simulink model "robot_rk"  (R2014b)
settings: Solver=ode45  StartTime=0.0  StopTime=10  FixedStep=1e-4  RelTol=1e-3
values from neighbouring files (symbols this model uses):
  robot_floor_friction_coeff = 0.6    [robot_init.m]
  robot_floor_position_gain = -1e5    (= -100000)    [robot_init.m]
  robot_floor_speed_gain = -1e3    (= -1000)    [robot_init.m]
  robot_gravity = [0 0 -9.80665]    [robot_init.m]
undefined symbols (not defined in the file or in its folder): CM730_acc_center, CM730_acc_gain, CM730_default, CM730_gyro_center, CM730_gyro_gain, CM730_sample_time, FSR_max, FSR_no_load, FSR_sample_time, FSR_scale, MX28_default, MX28_inertia, MX28_Te, X, Y, Z
libraries: sm_lib x158, fl_lib x128, nesl_utility x77
(part 4 of 6)

== system robot_rk/Right Leg/Right Ankle Pitch (15) ==
  Inertia : sm_lib/Body Elements/Inertia  InertiaType=Custom  Mass=1  MassUnits=g  CenterOfMass=[0 0 0]  CenterOfMassUnits=m  MomentsOfInertia=[0 0 MX28_inertia]  MomentsOfInertiaUnits=kg*m^2  ProductsOfInertia=[0 0 0]  ProductsOfInertiaUnits=kg*m^2  BlockFunction=simmechanics.library.body_elements.inertia
  MX28 Command : DataStoreRead  DataStoreName=MX28_ID15  SampleTime=MX28_Te  DataStoreElements=MX28_ID15.CW_angle_limit#MX28_ID15.CCW_angle_limit#MX28_ID15.torque_enable#MX28_ID15.D_gain#MX28_ID15.I_gain#MX28_ID15.P_gain#MX28_ID15.goal_position#MX28_ID15.moving_speed#MX28_ID15.torque_limit
  MX28 State : DataStoreWrite  DataStoreName=MX28_ID15  DataStoreElements=MX28_ID15.present_position#MX28_ID15.present_speed#MX28_ID15.present_load#MX28_ID15.moving#MX28_ID15.pwm
  Model : ModelReference  ModelNameDialog=MX28.slx  SimulationMode=Normal  ModelReferenceVersion=1.66  CopyOfModelName=MX28.slx  DefaultDataLogging=on
  Position converter : nesl_utility/PS-Simulink Converter  PhysicalDomain=network_engine_domain  SubClassName=ps_output  LeftPortType=input  RightPortType=output  PseudoPeriodic=off  Frequencies=[]  Unit=rad  AffineConversion=off
  Revolute Joint : sm_lib/Joints/Revolute Joint  SenseConstraintForce=off  SenseConstraintForceX=off  SenseConstraintForceY=off  SenseConstraintForceZ=off  SenseConstraintTorque=off  SenseConstraintTorqueX=off  SenseConstraintTorqueY=off  SenseConstraintTorqueZ=off  SenseTotalForce=off  SenseTotalForceX=off  SenseTotalForceY=off  SenseTotalForceZ=off  SenseTotalTorque=off  SenseTotalTorqueX=off  SenseTotalTorqueY=off  SenseTotalTorqueZ=off  CompositeWrenchDir=FollowerOnBase  CompositeWrenchFrame=BaseFrame  EquilibriumPosition=0  EquilibriumPositionUnits=deg  SpringStiffness=0  SpringStiffnessUnits=N*m/deg  DampingCoefficient=MX28_lub_friction  DampingCoefficientUnits=N*m/(rad/s)  TorqueActuationMode=InputTorque  MotionActuationMode=ComputedMotion  SensePosition=on  SenseVelocity=on  SenseAcceleration=off  SenseTorqueForce=off  PositionTargetValue=MX28_init_position  PositionTargetValueUnits=rad  PositionTargetSpecify=on  PositionTargetPriority=High  VelocityTargetValue=MX28_init_speed  VelocityTargetValueUnits=rad/s  VelocityTargetSpecify=on  VelocityTargetPriority=High  BlockFunction=simmechanics.library.joints.revolute_joint
  Speed converter : nesl_utility/PS-Simulink Converter  PhysicalDomain=network_engine_domain  SubClassName=ps_output  LeftPortType=input  RightPortType=output  PseudoPeriodic=off  Frequencies=[]  Unit=rad/s  AffineConversion=off
  Torque converter : nesl_utility/Simulink-PS Converter  PhysicalDomain=network_engine_domain  SubClassName=ps_input  LeftPortType=input  RightPortType=output  PseudoPeriodic=off  Frequencies=[]  NoiseDistribution=none  NoiseParameters=[]  Unit=N*m  AffineConversion=off  InputFiltering=off  SimscapeFilterOrder=1  InputFilterTimeConstant=0.001  UdotUserProvided=1
  Base : PMIOPort  Port=1  Side=Left
  Axis : PMIOPort  Port=2  Side=Right
  wires:
  Model/4 -> MX28 State/3
  Model/2 -> MX28 State/1
  Model/5 -> MX28 State/4
  Model/3 -> MX28 State/2
  MX28 Command/3 -> Model/5
  MX28 Command/6 -> Model/8
  MX28 Command/4 -> Model/6
  MX28 Command/5 -> Model/7
  MX28 Command/7 -> Model/9
  MX28 Command/2 -> Model/4
  MX28 Command/1 -> Model/3
  Position converter/1 -> Model/2
  Speed converter/1 -> Model/1
  Model/1 -> Torque converter/1
  Model/6 -> MX28 State/5
  MX28 Command/8 -> Model/10
  MX28 Command/9 -> Model/11
  connections:
  Axis/RConn1 -- Revolute Joint/RConn1 -- Inertia/RConn1
  Revolute Joint/LConn1 -- Base/RConn1
  Revolute Joint/RConn3 -- Speed converter/LConn1
  Revolute Joint/RConn2 -- Position converter/LConn1
  Revolute Joint/LConn2 -- Torque converter/RConn1

== system robot_rk/Right Leg/Right Ankle Roll (17) ==
  Inertia : sm_lib/Body Elements/Inertia  InertiaType=Custom  Mass=1  MassUnits=g  CenterOfMass=[0 0 0]  CenterOfMassUnits=m  MomentsOfInertia=[0 0 MX28_inertia]  MomentsOfInertiaUnits=kg*m^2  ProductsOfInertia=[0 0 0]  ProductsOfInertiaUnits=kg*m^2  BlockFunction=simmechanics.library.body_elements.inertia
  MX28 Command : DataStoreRead  DataStoreName=MX28_ID17  SampleTime=MX28_Te  DataStoreElements=MX28_ID17.CW_angle_limit#MX28_ID17.CCW_angle_limit#MX28_ID17.torque_enable#MX28_ID17.D_gain#MX28_ID17.I_gain#MX28_ID17.P_gain#MX28_ID17.goal_position#MX28_ID17.moving_speed#MX28_ID17.torque_limit
  MX28 State : DataStoreWrite  DataStoreName=MX28_ID17  DataStoreElements=MX28_ID17.present_position#MX28_ID17.present_speed#MX28_ID17.present_load#MX28_ID17.moving#MX28_ID17.pwm
  Model : ModelReference  ModelNameDialog=MX28.slx  SimulationMode=Normal  ModelReferenceVersion=1.66  CopyOfModelName=MX28.slx  DefaultDataLogging=on
  Position converter : nesl_utility/PS-Simulink Converter  PhysicalDomain=network_engine_domain  SubClassName=ps_output  LeftPortType=input  RightPortType=output  PseudoPeriodic=off  Frequencies=[]  Unit=rad  AffineConversion=off
  Revolute Joint : sm_lib/Joints/Revolute Joint  SenseConstraintForce=off  SenseConstraintForceX=off  SenseConstraintForceY=off  SenseConstraintForceZ=off  SenseConstraintTorque=off  SenseConstraintTorqueX=off  SenseConstraintTorqueY=off  SenseConstraintTorqueZ=off  SenseTotalForce=off  SenseTotalForceX=off  SenseTotalForceY=off  SenseTotalForceZ=off  SenseTotalTorque=off  SenseTotalTorqueX=off  SenseTotalTorqueY=off  SenseTotalTorqueZ=off  CompositeWrenchDir=FollowerOnBase  CompositeWrenchFrame=BaseFrame  EquilibriumPosition=0  EquilibriumPositionUnits=deg  SpringStiffness=0  SpringStiffnessUnits=N*m/deg  DampingCoefficient=MX28_lub_friction  DampingCoefficientUnits=N*m/(rad/s)  TorqueActuationMode=InputTorque  MotionActuationMode=ComputedMotion  SensePosition=on  SenseVelocity=on  SenseAcceleration=off  SenseTorqueForce=off  PositionTargetValue=MX28_init_position  PositionTargetValueUnits=rad  PositionTargetSpecify=on  PositionTargetPriority=High  VelocityTargetValue=MX28_init_speed  VelocityTargetValueUnits=rad/s  VelocityTargetSpecify=on  VelocityTargetPriority=High  BlockFunction=simmechanics.library.joints.revolute_joint
  Speed converter : nesl_utility/PS-Simulink Converter  PhysicalDomain=network_engine_domain  SubClassName=ps_output  LeftPortType=input  RightPortType=output  PseudoPeriodic=off  Frequencies=[]  Unit=rad/s  AffineConversion=off
  Torque converter : nesl_utility/Simulink-PS Converter  PhysicalDomain=network_engine_domain  SubClassName=ps_input  LeftPortType=input  RightPortType=output  PseudoPeriodic=off  Frequencies=[]  NoiseDistribution=none  NoiseParameters=[]  Unit=N*m  AffineConversion=off  InputFiltering=off  SimscapeFilterOrder=1  InputFilterTimeConstant=0.001  UdotUserProvided=1
  Base : PMIOPort  Port=1  Side=Left
  Axis : PMIOPort  Port=2  Side=Right
  wires:
  Model/4 -> MX28 State/3
  Model/2 -> MX28 State/1
  Model/5 -> MX28 State/4
  Model/3 -> MX28 State/2
  MX28 Command/3 -> Model/5
  MX28 Command/6 -> Model/8
  MX28 Command/4 -> Model/6
  MX28 Command/5 -> Model/7
  MX28 Command/7 -> Model/9
  MX28 Command/2 -> Model/4
  MX28 Command/1 -> Model/3
  Position converter/1 -> Model/2
  Speed converter/1 -> Model/1
  Model/1 -> Torque converter/1
  Model/6 -> MX28 State/5
  MX28 Command/8 -> Model/10
  MX28 Command/9 -> Model/11
  connections:
  Axis/RConn1 -- Revolute Joint/RConn1 -- Inertia/RConn1
  Revolute Joint/LConn1 -- Base/RConn1
  Revolute Joint/RConn3 -- Speed converter/LConn1
  Revolute Joint/RConn2 -- Position converter/LConn1
  Revolute Joint/LConn2 -- Torque converter/RConn1

== system robot_rk/Right Leg/Right Foot ==
  Right Foot Axis to Back Left : sm_lib/Frames and Transforms/Rigid Transform  TranslationMethod=Cartesian  TranslationLengthUnit=mm  TranslationStandardAxis=+Z  TranslationStandardOffset=0  TranslationCartesianOffset=[-14.5 33.5 -28.9]  TranslationROffset=0  TranslationROffsetUnits=m  TranslationZOffset=0  TranslationZOffsetUnits=m  TranslationThetaOffset=0  TranslationThetaOffsetUnits=deg  RotationMethod=AlignedAxes  RotationAngleUnits=deg  RotationStandardAxis=+Z  RotationAngle=0.0  RotationArbitraryAxis=[0 0 1]  FollAlignAxisA=+X  BaseAlignAxisA=-X  FollAlignAxisB=+Z  BaseAlignAxisB=-Y  RotationMatrix=[1 0 0; 0 1 0; 0 0 1]  BlockFunction=simmechanics.library.frames_transforms.rigid_transform
  Right Foot Axis to Back Right : sm_lib/Frames and Transforms/Rigid Transform  TranslationMethod=Cartesian  TranslationLengthUnit=mm  TranslationStandardAxis=+Z  TranslationStandardOffset=0  TranslationCartesianOffset=[35.5 33.5 -28.9]  TranslationROffset=0  TranslationROffsetUnits=m  TranslationZOffset=0  TranslationZOffsetUnits=m  TranslationThetaOffset=0  TranslationThetaOffsetUnits=deg  RotationMethod=AlignedAxes  RotationAngleUnits=deg  RotationStandardAxis=+Z  RotationAngle=0.0  RotationArbitraryAxis=[0 0 1]  FollAlignAxisA=+X  BaseAlignAxisA=-X  FollAlignAxisB=+Z  BaseAlignAxisB=-Y  RotationMatrix=[1 0 0; 0 1 0; 0 0 1]  BlockFunction=simmechanics.library.frames_transforms.rigid_transform
  Right Foot Axis to Front Left : sm_lib/Frames and Transforms/Rigid Transform  TranslationMethod=Cartesian  TranslationLengthUnit=mm  TranslationStandardAxis=+Z  TranslationStandardOffset=0  TranslationCartesianOffset=[-14.5 33.5 73.1]  TranslationROffset=0  TranslationROffsetUnits=m  TranslationZOffset=0  TranslationZOffsetUnits=m  TranslationThetaOffset=0  TranslationThetaOffsetUnits=deg  RotationMethod=AlignedAxes  RotationAngleUnits=deg  RotationStandardAxis=+Z  RotationAngle=0.0  RotationArbitraryAxis=[0 0 1]  FollAlignAxisA=+X  BaseAlignAxisA=-X  FollAlignAxisB=+Z  BaseAlignAxisB=-Y  RotationMatrix=[1 0 0; 0 1 0; 0 0 1]  BlockFunction=simmechanics.library.frames_transforms.rigid_transform
  Right Foot Axis to Front Right : sm_lib/Frames and Transforms/Rigid Transform  TranslationMethod=Cartesian  TranslationLengthUnit=mm  TranslationStandardAxis=+Z  TranslationStandardOffset=0  TranslationCartesianOffset=[35.5 33.5 73.1]  TranslationROffset=0  TranslationROffsetUnits=m  TranslationZOffset=0  TranslationZOffsetUnits=m  TranslationThetaOffset=0  TranslationThetaOffsetUnits=deg  RotationMethod=AlignedAxes  RotationAngleUnits=deg  RotationStandardAxis=+Z  RotationAngle=0.0  RotationArbitraryAxis=[0 0 1]  FollAlignAxisA=+X  BaseAlignAxisA=-X  FollAlignAxisB=+Z  BaseAlignAxisB=-Y  RotationMatrix=[1 0 0; 0 1 0; 0 0 1]  BlockFunction=simmechanics.library.frames_transforms.rigid_transform
  Solid : sm_lib/Body Elements/Solid  InertiaType=Custom  Mass=76.78  MassUnits=g  CenterOfMass=[7.76 24.5 17.25]  CenterOfMassUnits=mm  MomentsOfInertia=[69069 85303 36676]  MomentsOfInertiaUnits=g*mm^2  ProductsOfInertia=[4062 778 2754]  ProductsOfInertiaUnits=g*mm^2  DensityBased=on  Density=1000  DensityUnits=kg/(m^3)  GraphicType=FromGeometry  MarkerShape=Sphere  MarkerSize=10  MarkerSizeUnits=m  GraphicVisPropType=SimpleVisualProperties  GraphicDiffuseColor=[0.5 0.5 0.5]  GraphicSpecularColor=[0.5 0.5 0.5 1.0]  GraphicAmbientColor=[0.15 0.15 0.15 1.0]  GraphicEmissiveColor=[0.0 0.0 0.0 1.0]  GraphicShininess=75  GraphicOpacity=1.0  GeometryShape=FromFile  RectangleSize=[1 1]  RectangleSizeUnits=m  BrickDimensions=[1 1 1]  BrickDimensionUnits=m  CylinderRadius=1  CylinderRadiusUnits=m  CylinderLength=1  CylinderLengthUnits=m  SphereRadius=1  SphereRadiusUnits=m  EllipsoidRadii=[1 1 1]  EllipsoidRadiiUnits=m  ExtrusionCrossSection=[1 1; -1 1; -1 -1; 1 -1]  ExtrusionCrossSectionUnits=m  ExtrusionLength=1  ExtrusionLengthUnits=m  PolygonNumSides=3  PolygonOuterRadius=1  PolygonOuterRadiusUnits=m  ExtGeomFileType=STL  ExtGeomFileName=D:\Ker Lann\systemes\darwin\kinematics\STL\Right_Foot.STL  ExtGeomFileUnits=mm  RevolutionCrossSection=[1 1; 1 -1; 2 -1; 2 1]  RevolutionCrossSectionUnits=m  RevolutionExtent=Full  RevolutionAngle=180  RevolutionAngleUnits=deg  BlockFunction=simmechanics.library.body_elements.solid
  Right Ankle Roll : PMIOPort  Port=1  Side=Left
  Front Left : PMIOPort  Port=2  Side=Right
  Front Right : PMIOPort  Port=3  Side=Right
  Back Right : PMIOPort  Port=4  Side=Right
  Back Left : PMIOPort  Port=5  Side=Right
  connections:
  Right Foot Axis to Front Left/LConn1 -- Right Foot Axis to Back Right/LConn1 -- Solid/RConn1 -- Right Ankle Roll/RConn1 -- Right Foot Axis to Back Left/LConn1 -- Right Foot Axis to Front Right/LConn1
  Front Left/RConn1 -- Right Foot Axis to Front Left/RConn1
  Back Right/RConn1 -- Right Foot Axis to Back Right/RConn1
  Front Right/RConn1 -- Right Foot Axis to Front Right/RConn1
  Back Left/RConn1 -- Right Foot Axis to Back Left/RConn1

== system robot_rk/Right Leg/Right Hip Pitch (11) ==
  Inertia : sm_lib/Body Elements/Inertia  InertiaType=Custom  Mass=1  MassUnits=g  CenterOfMass=[0 0 0]  CenterOfMassUnits=m  MomentsOfInertia=[0 0 MX28_inertia]  MomentsOfInertiaUnits=kg*m^2  ProductsOfInertia=[0 0 0]  ProductsOfInertiaUnits=kg*m^2  BlockFunction=simmechanics.library.body_elements.inertia
  MX28 Command : DataStoreRead  DataStoreName=MX28_ID11  SampleTime=MX28_Te  DataStoreElements=MX28_ID11.CW_angle_limit#MX28_ID11.CCW_angle_limit#MX28_ID11.torque_enable#MX28_ID11.D_gain#MX28_ID11.I_gain#MX28_ID11.P_gain#MX28_ID11.goal_position#MX28_ID11.moving_speed#MX28_ID11.torque_limit
  MX28 State : DataStoreWrite  DataStoreName=MX28_ID11  DataStoreElements=MX28_ID11.present_position#MX28_ID11.present_speed#MX28_ID11.present_load#MX28_ID11.moving#MX28_ID11.pwm
  Model : ModelReference  ModelNameDialog=MX28.slx  SimulationMode=Normal  ModelReferenceVersion=1.66  CopyOfModelName=MX28.slx  DefaultDataLogging=on
  Position converter : nesl_utility/PS-Simulink Converter  PhysicalDomain=network_engine_domain  SubClassName=ps_output  LeftPortType=input  RightPortType=output  PseudoPeriodic=off  Frequencies=[]  Unit=rad  AffineConversion=off
  Revolute Joint : sm_lib/Joints/Revolute Joint  SenseConstraintForce=off  SenseConstraintForceX=off  SenseConstraintForceY=off  SenseConstraintForceZ=off  SenseConstraintTorque=off  SenseConstraintTorqueX=off  SenseConstraintTorqueY=off  SenseConstraintTorqueZ=off  SenseTotalForce=off  SenseTotalForceX=off  SenseTotalForceY=off  SenseTotalForceZ=off  SenseTotalTorque=off  SenseTotalTorqueX=off  SenseTotalTorqueY=off  SenseTotalTorqueZ=off  CompositeWrenchDir=FollowerOnBase  CompositeWrenchFrame=BaseFrame  EquilibriumPosition=0  EquilibriumPositionUnits=deg  SpringStiffness=0  SpringStiffnessUnits=N*m/deg  DampingCoefficient=MX28_lub_friction  DampingCoefficientUnits=N*m/(rad/s)  TorqueActuationMode=InputTorque  MotionActuationMode=ComputedMotion  SensePosition=on  SenseVelocity=on  SenseAcceleration=off  SenseTorqueForce=off  PositionTargetValue=MX28_init_position  PositionTargetValueUnits=rad  PositionTargetSpecify=on  PositionTargetPriority=High  VelocityTargetValue=MX28_init_speed  VelocityTargetValueUnits=rad/s  VelocityTargetSpecify=on  VelocityTargetPriority=High  BlockFunction=simmechanics.library.joints.revolute_joint
  Speed converter : nesl_utility/PS-Simulink Converter  PhysicalDomain=network_engine_domain  SubClassName=ps_output  LeftPortType=input  RightPortType=output  PseudoPeriodic=off  Frequencies=[]  Unit=rad/s  AffineConversion=off
  Torque converter : nesl_utility/Simulink-PS Converter  PhysicalDomain=network_engine_domain  SubClassName=ps_input  LeftPortType=input  RightPortType=output  PseudoPeriodic=off  Frequencies=[]  NoiseDistribution=none  NoiseParameters=[]  Unit=N*m  AffineConversion=off  InputFiltering=off  SimscapeFilterOrder=1  InputFilterTimeConstant=0.001  UdotUserProvided=1
  Base : PMIOPort  Port=1  Side=Left
  Axis : PMIOPort  Port=2  Side=Right
  wires:
  Model/4 -> MX28 State/3
  Model/2 -> MX28 State/1
  Model/5 -> MX28 State/4
  Model/3 -> MX28 State/2
  MX28 Command/3 -> Model/5
  MX28 Command/6 -> Model/8
  MX28 Command/4 -> Model/6
  MX28 Command/5 -> Model/7
  MX28 Command/7 -> Model/9
  MX28 Command/2 -> Model/4
  MX28 Command/1 -> Model/3
  Position converter/1 -> Model/2
  Speed converter/1 -> Model/1
  Model/1 -> Torque converter/1
  Model/6 -> MX28 State/5
  MX28 Command/8 -> Model/10
  MX28 Command/9 -> Model/11
  connections:
  Axis/RConn1 -- Revolute Joint/RConn1 -- Inertia/RConn1
  Revolute Joint/LConn1 -- Base/RConn1
  Revolute Joint/RConn3 -- Speed converter/LConn1
  Revolute Joint/RConn2 -- Position converter/LConn1
  Revolute Joint/LConn2 -- Torque converter/RConn1

== system robot_rk/Right Leg/Right Hip Roll ==
  Right Hip Roll Base to Right Hip Pitch Base : sm_lib/Frames and Transforms/Rigid Transform  TranslationMethod=Cartesian  TranslationLengthUnit=mm  TranslationStandardAxis=+Z  TranslationStandardOffset=0  TranslationCartesianOffset=[23.9 0 19.1]  TranslationROffset=0  TranslationROffsetUnits=m  TranslationZOffset=0  TranslationZOffsetUnits=m  TranslationThetaOffset=0  TranslationThetaOffsetUnits=deg  RotationMethod=AlignedAxes  RotationAngleUnits=deg  RotationStandardAxis=+Z  RotationAngle=0  RotationArbitraryAxis=[0 0 1]  FollAlignAxisA=+Z  BaseAlignAxisA=+X  FollAlignAxisB=+Y  BaseAlignAxisB=+Y  RotationMatrix=[1 0 0; 0 1 0; 0 0 1]  BlockFunction=simmechanics.library.frames_transforms.rigid_transform
  Solid : sm_lib/Body Elements/Solid  InertiaType=Custom  Mass=166.79  MassUnits=g  CenterOfMass=[-0.21 -11.21 1.04]  CenterOfMassUnits=mm  MomentsOfInertia=[11817 12213 6949]  MomentsOfInertiaUnits=g*mm^2  ProductsOfInertia=[4006 104 -199]  ProductsOfInertiaUnits=g*mm^2  DensityBased=on  Density=1000  DensityUnits=kg/(m^3)  GraphicType=FromGeometry  MarkerShape=Sphere  MarkerSize=10  MarkerSizeUnits=m  GraphicVisPropType=SimpleVisualProperties  GraphicDiffuseColor=[0.5 0.5 0.5]  GraphicSpecularColor=[0.5 0.5 0.5 1.0]  GraphicAmbientColor=[0.15 0.15 0.15 1.0]  GraphicEmissiveColor=[0.0 0.0 0.0 1.0]  GraphicShininess=75  GraphicOpacity=1.0  GeometryShape=FromFile  RectangleSize=[1 1]  RectangleSizeUnits=m  BrickDimensions=[1 1 1]  BrickDimensionUnits=mm  CylinderRadius=1  CylinderRadiusUnits=m  CylinderLength=1  CylinderLengthUnits=m  SphereRadius=1  SphereRadiusUnits=m  EllipsoidRadii=[1 1 1]  EllipsoidRadiiUnits=m  ExtrusionCrossSection=[1 1; -1 1; -1 -1; 1 -1]  ExtrusionCrossSectionUnits=m  ExtrusionLength=1  ExtrusionLengthUnits=m  PolygonNumSides=3  PolygonOuterRadius=1  PolygonOuterRadiusUnits=m  ExtGeomFileType=STL  ExtGeomFileName=D:\Ker Lann\systemes\darwin\kinematics\STL\Right_Hip2.STL  ExtGeomFileUnits=mm  RevolutionCrossSection=[1 1; 1 -1; 2 -1; 2 1]  RevolutionCrossSectionUnits=m  RevolutionExtent=Full  RevolutionAngle=180  RevolutionAngleUnits=deg  BlockFunction=simmechanics.library.body_elements.solid
  Right Hip Roll : PMIOPort  Port=1  Side=Left
  Right Hip Pitch : PMIOPort  Port=2  Side=Right
  connections:
  Right Hip Roll Base to Right Hip Pitch Base/LConn1 -- Solid/RConn1 -- Right Hip Roll/RConn1
  Right Hip Roll Base to Right Hip Pitch Base/RConn1 -- Right Hip Pitch/RConn1

== system robot_rk/Right Leg/Right Hip Roll (9) ==
  Inertia : sm_lib/Body Elements/Inertia  InertiaType=Custom  Mass=1  MassUnits=g  CenterOfMass=[0 0 0]  CenterOfMassUnits=m  MomentsOfInertia=[0 0 MX28_inertia]  MomentsOfInertiaUnits=kg*m^2  ProductsOfInertia=[0 0 0]  ProductsOfInertiaUnits=kg*m^2  BlockFunction=simmechanics.library.body_elements.inertia
  MX28 Command : DataStoreRead  DataStoreName=MX28_ID9  SampleTime=MX28_Te  DataStoreElements=MX28_ID9.CW_angle_limit#MX28_ID9.CCW_angle_limit#MX28_ID9.torque_enable#MX28_ID9.D_gain#MX28_ID9.I_gain#MX28_ID9.P_gain#MX28_ID9.goal_position#MX28_ID9.moving_speed#MX28_ID9.torque_limit
  MX28 State : DataStoreWrite  DataStoreName=MX28_ID9  DataStoreElements=MX28_ID9.present_position#MX28_ID9.present_speed#MX28_ID9.present_load#MX28_ID9.moving#MX28_ID9.pwm
  Model : ModelReference  ModelNameDialog=MX28.slx  SimulationMode=Normal  ModelReferenceVersion=1.66  CopyOfModelName=MX28.slx  DefaultDataLogging=on
  Position converter : nesl_utility/PS-Simulink Converter  PhysicalDomain=network_engine_domain  SubClassName=ps_output  LeftPortType=input  RightPortType=output  PseudoPeriodic=off  Frequencies=[]  Unit=rad  AffineConversion=off
  Revolute Joint : sm_lib/Joints/Revolute Joint  SenseConstraintForce=off  SenseConstraintForceX=off  SenseConstraintForceY=off  SenseConstraintForceZ=off  SenseConstraintTorque=off  SenseConstraintTorqueX=off  SenseConstraintTorqueY=off  SenseConstraintTorqueZ=off  SenseTotalForce=off  SenseTotalForceX=off  SenseTotalForceY=off  SenseTotalForceZ=off  SenseTotalTorque=off  SenseTotalTorqueX=off  SenseTotalTorqueY=off  SenseTotalTorqueZ=off  CompositeWrenchDir=FollowerOnBase  CompositeWrenchFrame=BaseFrame  EquilibriumPosition=0  EquilibriumPositionUnits=deg  SpringStiffness=0  SpringStiffnessUnits=N*m/deg  DampingCoefficient=MX28_lub_friction  DampingCoefficientUnits=N*m/(rad/s)  TorqueActuationMode=InputTorque  MotionActuationMode=ComputedMotion  SensePosition=on  SenseVelocity=on  SenseAcceleration=off  SenseTorqueForce=off  PositionTargetValue=MX28_init_position  PositionTargetValueUnits=rad  PositionTargetSpecify=on  PositionTargetPriority=High  VelocityTargetValue=MX28_init_speed  VelocityTargetValueUnits=rad/s  VelocityTargetSpecify=on  VelocityTargetPriority=High  BlockFunction=simmechanics.library.joints.revolute_joint
  Speed converter : nesl_utility/PS-Simulink Converter  PhysicalDomain=network_engine_domain  SubClassName=ps_output  LeftPortType=input  RightPortType=output  PseudoPeriodic=off  Frequencies=[]  Unit=rad/s  AffineConversion=off
  Torque converter : nesl_utility/Simulink-PS Converter  PhysicalDomain=network_engine_domain  SubClassName=ps_input  LeftPortType=input  RightPortType=output  PseudoPeriodic=off  Frequencies=[]  NoiseDistribution=none  NoiseParameters=[]  Unit=N*m  AffineConversion=off  InputFiltering=off  SimscapeFilterOrder=1  InputFilterTimeConstant=0.001  UdotUserProvided=1
  Base : PMIOPort  Port=1  Side=Left
  Axis : PMIOPort  Port=2  Side=Right
  wires:
  Model/4 -> MX28 State/3
  Model/2 -> MX28 State/1
  Model/5 -> MX28 State/4
  Model/3 -> MX28 State/2
  MX28 Command/3 -> Model/5
  MX28 Command/6 -> Model/8
  MX28 Command/4 -> Model/6
  MX28 Command/5 -> Model/7
  MX28 Command/7 -> Model/9
  MX28 Command/2 -> Model/4
  MX28 Command/1 -> Model/3
  Speed converter/1 -> Model/1
  Position converter/1 -> Model/2
  Model/1 -> Torque converter/1
  Model/6 -> MX28 State/5
  MX28 Command/8 -> Model/10
  MX28 Command/9 -> Model/11
  connections:
  Axis/RConn1 -- Revolute Joint/RConn1 -- Inertia/RConn1
  Revolute Joint/LConn1 -- Base/RConn1
  Revolute Joint/RConn3 -- Speed converter/LConn1
  Revolute Joint/RConn2 -- Position converter/LConn1
  Revolute Joint/LConn2 -- Torque converter/RConn1

== system robot_rk/Right Leg/Right Hip Yaw ==
  Right Hip Yaw Axis to Right Hip Roll Axis : sm_lib/Frames and Transforms/Rigid Transform  TranslationMethod=Cartesian  TranslationLengthUnit=mm  TranslationStandardAxis=+Z  TranslationStandardOffset=0  TranslationCartesianOffset=[24.85 0 28.35]  TranslationROffset=0  TranslationROffsetUnits=m  TranslationZOffset=0  TranslationZOffsetUnits=m  TranslationThetaOffset=0  TranslationThetaOffsetUnits=deg  RotationMethod=AlignedAxes  RotationAngleUnits=deg  RotationStandardAxis=+Z  RotationAngle=0  RotationArbitraryAxis=[0 0 1]  FollAlignAxisA=+Y  BaseAlignAxisA=+Z  FollAlignAxisB=+X  BaseAlignAxisB=-Y  RotationMatrix=[1 0 0; 0 1 0; 0 0 1]  BlockFunction=simmechanics.library.frames_transforms.rigid_transform
  Solid : sm_lib/Body Elements/Solid  InertiaType=Custom  Mass=34.1  MassUnits=g  CenterOfMass=[7.53 0 10.27]  CenterOfMassUnits=mm  MomentsOfInertia=[8263 18980 13482]  MomentsOfInertiaUnits=g*mm^2  ProductsOfInertia=[0 3667 0]  ProductsOfInertiaUnits=g*mm^2  DensityBased=on  Density=1000  DensityUnits=kg/(m^3)  GraphicType=FromGeometry  MarkerShape=Sphere  MarkerSize=10  MarkerSizeUnits=m  GraphicVisPropType=SimpleVisualProperties  GraphicDiffuseColor=[0.5 0.5 0.5]  GraphicSpecularColor=[0.5 0.5 0.5 1.0]  GraphicAmbientColor=[0.15 0.15 0.15 1.0]  GraphicEmissiveColor=[0.0 0.0 0.0 1.0]  GraphicShininess=75  GraphicOpacity=1.0  GeometryShape=FromFile  RectangleSize=[1 1]  RectangleSizeUnits=m  BrickDimensions=[1 1 1]  BrickDimensionUnits=mm  CylinderRadius=1  CylinderRadiusUnits=m  CylinderLength=1  CylinderLengthUnits=m  SphereRadius=1  SphereRadiusUnits=m  EllipsoidRadii=[1 1 1]  EllipsoidRadiiUnits=m  ExtrusionCrossSection=[1 1; -1 1; -1 -1; 1 -1]  ExtrusionCrossSectionUnits=m  ExtrusionLength=1  ExtrusionLengthUnits=m  PolygonNumSides=3  PolygonOuterRadius=1  PolygonOuterRadiusUnits=m  ExtGeomFileType=STL  ExtGeomFileName=D:\Ker Lann\systemes\darwin\kinematics\STL\Hip1.STL  ExtGeomFileUnits=mm  RevolutionCrossSection=[1 1; 1 -1; 2 -1; 2 1]  RevolutionCrossSectionUnits=m  RevolutionExtent=Full  RevolutionAngle=180  RevolutionAngleUnits=deg  BlockFunction=simmechanics.library.body_elements.solid
  Right Hip Yaw : PMIOPort  Port=1  Side=Left
  Right Hip Roll : PMIOPort  Port=2  Side=Right
  connections:
  Right Hip Yaw Axis to Right Hip Roll Axis/RConn1 -- Right Hip Roll/RConn1
  Solid/RConn1 -- Right Hip Yaw Axis to Right Hip Roll Axis/LConn1 -- Right Hip Yaw/RConn1

== system robot_rk/Right Leg/Right Hip Yaw (7) ==
  Inertia : sm_lib/Body Elements/Inertia  InertiaType=Custom  Mass=1  MassUnits=g  CenterOfMass=[0 0 0]  CenterOfMassUnits=m  MomentsOfInertia=[0 0 MX28_inertia]  MomentsOfInertiaUnits=kg*m^2  ProductsOfInertia=[0 0 0]  ProductsOfInertiaUnits=kg*m^2  BlockFunction=simmechanics.library.body_elements.inertia
  MX28 Command : DataStoreRead  DataStoreName=MX28_ID7  SampleTime=MX28_Te  DataStoreElements=MX28_ID7.CW_angle_limit#MX28_ID7.CCW_angle_limit#MX28_ID7.torque_enable#MX28_ID7.D_gain#MX28_ID7.I_gain#MX28_ID7.P_gain#MX28_ID7.goal_position#MX28_ID7.moving_speed#MX28_ID7.torque_limit
  MX28 State : DataStoreWrite  DataStoreName=MX28_ID7  DataStoreElements=MX28_ID7.present_position#MX28_ID7.present_speed#MX28_ID7.present_load#MX28_ID7.moving#MX28_ID7.pwm
  Model : ModelReference  ModelNameDialog=MX28.slx  SimulationMode=Normal  ModelReferenceVersion=1.66  CopyOfModelName=MX28.slx  DefaultDataLogging=on
  Position converter : nesl_utility/PS-Simulink Converter  PhysicalDomain=network_engine_domain  SubClassName=ps_output  LeftPortType=input  RightPortType=output  PseudoPeriodic=off  Frequencies=[]  Unit=rad  AffineConversion=off
  Revolute Joint : sm_lib/Joints/Revolute Joint  SenseConstraintForce=off  SenseConstraintForceX=off  SenseConstraintForceY=off  SenseConstraintForceZ=off  SenseConstraintTorque=off  SenseConstraintTorqueX=off  SenseConstraintTorqueY=off  SenseConstraintTorqueZ=off  SenseTotalForce=off  SenseTotalForceX=off  SenseTotalForceY=off  SenseTotalForceZ=off  SenseTotalTorque=off  SenseTotalTorqueX=off  SenseTotalTorqueY=off  SenseTotalTorqueZ=off  CompositeWrenchDir=FollowerOnBase  CompositeWrenchFrame=BaseFrame  EquilibriumPosition=0  EquilibriumPositionUnits=deg  SpringStiffness=0  SpringStiffnessUnits=N*m/deg  DampingCoefficient=MX28_lub_friction  DampingCoefficientUnits=N*m/(rad/s)  TorqueActuationMode=InputTorque  MotionActuationMode=ComputedMotion  SensePosition=on  SenseVelocity=on  SenseAcceleration=off  SenseTorqueForce=off  PositionTargetValue=MX28_init_position  PositionTargetValueUnits=rad  PositionTargetSpecify=on  PositionTargetPriority=High  VelocityTargetValue=MX28_init_speed  VelocityTargetValueUnits=rad/s  VelocityTargetSpecify=on  VelocityTargetPriority=High  BlockFunction=simmechanics.library.joints.revolute_joint
  Speed converter : nesl_utility/PS-Simulink Converter  PhysicalDomain=network_engine_domain  SubClassName=ps_output  LeftPortType=input  RightPortType=output  PseudoPeriodic=off  Frequencies=[]  Unit=rad/s  AffineConversion=off
  Torque converter : nesl_utility/Simulink-PS Converter  PhysicalDomain=network_engine_domain  SubClassName=ps_input  LeftPortType=input  RightPortType=output  PseudoPeriodic=off  Frequencies=[]  NoiseDistribution=none  NoiseParameters=[]  Unit=N*m  AffineConversion=off  InputFiltering=off  SimscapeFilterOrder=1  InputFilterTimeConstant=0.001  UdotUserProvided=1
  Base : PMIOPort  Port=1  Side=Left
  Axis : PMIOPort  Port=2  Side=Right
  wires:
  Model/4 -> MX28 State/3
  Model/2 -> MX28 State/1
  Model/5 -> MX28 State/4
  Model/3 -> MX28 State/2
  MX28 Command/3 -> Model/5
  MX28 Command/6 -> Model/8
  MX28 Command/4 -> Model/6
  MX28 Command/5 -> Model/7
  MX28 Command/7 -> Model/9
  MX28 Command/2 -> Model/4
  MX28 Command/1 -> Model/3
  Speed converter/1 -> Model/1
  Position converter/1 -> Model/2
  Model/1 -> Torque converter/1
  Model/6 -> MX28 State/5
  MX28 Command/8 -> Model/10
  MX28 Command/9 -> Model/11
  connections:
  Axis/RConn1 -- Revolute Joint/RConn1 -- Inertia/RConn1
  Revolute Joint/LConn1 -- Base/RConn1
  Revolute Joint/RConn3 -- Speed converter/LConn1
  Revolute Joint/RConn2 -- Position converter/LConn1
  Revolute Joint/LConn2 -- Torque converter/RConn1

== system robot_rk/Right Leg/Right Knee (13) ==
  Inertia : sm_lib/Body Elements/Inertia  InertiaType=Custom  Mass=1  MassUnits=g  CenterOfMass=[0 0 0]  CenterOfMassUnits=m  MomentsOfInertia=[0 0 MX28_inertia]  MomentsOfInertiaUnits=kg*m^2  ProductsOfInertia=[0 0 0]  ProductsOfInertiaUnits=kg*m^2  BlockFunction=simmechanics.library.body_elements.inertia
  MX28 Command : DataStoreRead  DataStoreName=MX28_ID13  SampleTime=MX28_Te  DataStoreElements=MX28_ID13.CW_angle_limit#MX28_ID13.CCW_angle_limit#MX28_ID13.torque_enable#MX28_ID13.D_gain#MX28_ID13.I_gain#MX28_ID13.P_gain#MX28_ID13.goal_position#MX28_ID13.moving_speed#MX28_ID13.torque_limit
  MX28 State : DataStoreWrite  DataStoreName=MX28_ID13  DataStoreElements=MX28_ID13.present_position#MX28_ID13.present_speed#MX28_ID13.present_load#MX28_ID13.moving#MX28_ID13.pwm
  Model : ModelReference  ModelNameDialog=MX28.slx  SimulationMode=Normal  ModelReferenceVersion=1.66  CopyOfModelName=MX28.slx  DefaultDataLogging=on
  Position converter : nesl_utility/PS-Simulink Converter  PhysicalDomain=network_engine_domain  SubClassName=ps_output  LeftPortType=input  RightPortType=output  PseudoPeriodic=off  Frequencies=[]  Unit=rad  AffineConversion=off
  Revolute Joint : sm_lib/Joints/Revolute Joint  SenseConstraintForce=off  SenseConstraintForceX=off  SenseConstraintForceY=off  SenseConstraintForceZ=off  SenseConstraintTorque=off  SenseConstraintTorqueX=off  SenseConstraintTorqueY=off  SenseConstraintTorqueZ=off  SenseTotalForce=off  SenseTotalForceX=off  SenseTotalForceY=off  SenseTotalForceZ=off  SenseTotalTorque=off  SenseTotalTorqueX=off  SenseTotalTorqueY=off  SenseTotalTorqueZ=off  CompositeWrenchDir=FollowerOnBase  CompositeWrenchFrame=BaseFrame  EquilibriumPosition=0  EquilibriumPositionUnits=deg  SpringStiffness=0  SpringStiffnessUnits=N*m/deg  DampingCoefficient=MX28_lub_friction  DampingCoefficientUnits=N*m/(rad/s)  TorqueActuationMode=InputTorque  MotionActuationMode=ComputedMotion  SensePosition=on  SenseVelocity=on  SenseAcceleration=off  SenseTorqueForce=off  PositionTargetValue=MX28_init_position  PositionTargetValueUnits=rad  PositionTargetSpecify=on  PositionTargetPriority=High  VelocityTargetValue=MX28_init_speed  VelocityTargetValueUnits=rad/s  VelocityTargetSpecify=on  VelocityTargetPriority=High  BlockFunction=simmechanics.library.joints.revolute_joint
  Speed converter : nesl_utility/PS-Simulink Converter  PhysicalDomain=network_engine_domain  SubClassName=ps_output  LeftPortType=input  RightPortType=output  PseudoPeriodic=off  Frequencies=[]  Unit=rad/s  AffineConversion=off
  Torque converter : nesl_utility/Simulink-PS Converter  PhysicalDomain=network_engine_domain  SubClassName=ps_input  LeftPortType=input  RightPortType=output  PseudoPeriodic=off  Frequencies=[]  NoiseDistribution=none  NoiseParameters=[]  Unit=N*m  AffineConversion=off  InputFiltering=off  SimscapeFilterOrder=1  InputFilterTimeConstant=0.001  UdotUserProvided=1
  Base : PMIOPort  Port=1  Side=Left
  Axis : PMIOPort  Port=2  Side=Right
  wires:
  Model/4 -> MX28 State/3
  Model/2 -> MX28 State/1
  Model/5 -> MX28 State/4
  Model/3 -> MX28 State/2
  MX28 Command/3 -> Model/5
  MX28 Command/6 -> Model/8
  MX28 Command/4 -> Model/6
  MX28 Command/5 -> Model/7
  MX28 Command/7 -> Model/9
  MX28 Command/2 -> Model/4
  MX28 Command/1 -> Model/3
  Position converter/1 -> Model/2
  Speed converter/1 -> Model/1
  Model/1 -> Torque converter/1
  Model/6 -> MX28 State/5
  MX28 Command/8 -> Model/10
  MX28 Command/9 -> Model/11
  connections:
  Axis/RConn1 -- Revolute Joint/RConn1 -- Inertia/RConn1
  Revolute Joint/LConn1 -- Base/RConn1
  Revolute Joint/RConn3 -- Speed converter/LConn1
  Revolute Joint/RConn2 -- Position converter/LConn1
  Revolute Joint/LConn2 -- Torque converter/RConn1

== system robot_rk/Right Leg/Right Lower Leg ==
  Right Lower Leg Axis to Right Ankle Axis : sm_lib/Frames and Transforms/Rigid Transform  TranslationMethod=Cartesian  TranslationLengthUnit=mm  TranslationStandardAxis=+Z  TranslationStandardOffset=0  TranslationCartesianOffset=[0 -93 0]  TranslationROffset=0  TranslationROffsetUnits=m  TranslationZOffset=0  TranslationZOffsetUnits=m  TranslationThetaOffset=0  TranslationThetaOffsetUnits=deg  RotationMethod=None  RotationAngleUnits=deg  RotationStandardAxis=+Z  RotationAngle=0  RotationArbitraryAxis=[0 0 1]  FollAlignAxisA=+X  BaseAlignAxisA=+Y  FollAlignAxisB=+Y  BaseAlignAxisB=+Z  RotationMatrix=[1 0 0; 0 1 0; 0 0 1]  BlockFunction=simmechanics.library.frames_transforms.rigid_transform
  Solid : sm_lib/Body Elements/Solid  InertiaType=Custom  Mass=76.54  MassUnits=g  CenterOfMass=[-6.06 -39.28 -19.71]  CenterOfMassUnits=mm  MomentsOfInertia=[129653 47800 108913]  MomentsOfInertiaUnits=g*mm^2  ProductsOfInertia=[-2435 1869 -13233]  ProductsOfInertiaUnits=g*mm^2  DensityBased=on  Density=1000  DensityUnits=kg/(m^3)  GraphicType=FromGeometry  MarkerShape=Sphere  MarkerSize=10  MarkerSizeUnits=m  GraphicVisPropType=SimpleVisualProperties  GraphicDiffuseColor=[0.5 0.5 0.5]  GraphicSpecularColor=[0.5 0.5 0.5 1.0]  GraphicAmbientColor=[0.15 0.15 0.15 1.0]  GraphicEmissiveColor=[0.0 0.0 0.0 1.0]  GraphicShininess=75  GraphicOpacity=1.0  GeometryShape=FromFile  RectangleSize=[1 1]  RectangleSizeUnits=m  BrickDimensions=[1 1 1]  BrickDimensionUnits=m  CylinderRadius=1  CylinderRadiusUnits=m  CylinderLength=1  CylinderLengthUnits=m  SphereRadius=1  SphereRadiusUnits=m  EllipsoidRadii=[1 1 1]  EllipsoidRadiiUnits=m  ExtrusionCrossSection=[1 1; -1 1; -1 -1; 1 -1]  ExtrusionCrossSectionUnits=m  ExtrusionLength=1  ExtrusionLengthUnits=m  PolygonNumSides=3  PolygonOuterRadius=1  PolygonOuterRadiusUnits=m  ExtGeomFileType=STL  ExtGeomFileName=D:\Ker Lann\systemes\darwin\kinematics\STL\Right_Lower_Leg.STL  ExtGeomFileUnits=mm  RevolutionCrossSection=[1 1; 1 -1; 2 -1; 2 1]  RevolutionCrossSectionUnits=m  RevolutionExtent=Full  RevolutionAngle=180  RevolutionAngleUnits=deg  BlockFunction=simmechanics.library.body_elements.solid
  Right Knee : PMIOPort  Port=1  Side=Left
  Right Ankle Pitch : PMIOPort  Port=2  Side=Right
  connections:
  Solid/RConn1 -- Right Lower Leg Axis to Right Ankle Axis/LConn1 -- Right Knee/RConn1
  Right Ankle Pitch/RConn1 -- Right Lower Leg Axis to Right Ankle Axis/RConn1

== system robot_rk/Right Leg/Right Thigh ==
  Right Hip Pitch Axis to Right Lower Leg Base : sm_lib/Frames and Transforms/Rigid Transform  TranslationMethod=Cartesian  TranslationLengthUnit=mm  TranslationStandardAxis=+Z  TranslationStandardOffset=0  TranslationCartesianOffset=[0 93 -1.75]  TranslationROffset=0  TranslationROffsetUnits=m  TranslationZOffset=0  TranslationZOffsetUnits=m  TranslationThetaOffset=0  TranslationThetaOffsetUnits=deg  RotationMethod=None  RotationAngleUnits=deg  RotationStandardAxis=+Z  RotationAngle=0  RotationArbitraryAxis=[0 0 1]  FollAlignAxisA=+X  BaseAlignAxisA=+Y  FollAlignAxisB=+Y  BaseAlignAxisB=+Z  RotationMatrix=[1 0 0; 0 1 0; 0 0 1]  BlockFunction=simmechanics.library.frames_transforms.rigid_transform
  Solid : sm_lib/Body Elements/Solid  InertiaType=Custom  Mass=120.35  MassUnits=g  CenterOfMass=[0.84 62.83 -22.82]  CenterOfMassUnits=mm  MomentsOfInertia=[55245 22027 41171]  MomentsOfInertiaUnits=g*mm^2  ProductsOfInertia=[-6442 -244 1518]  ProductsOfInertiaUnits=g*mm^2  DensityBased=on  Density=1000  DensityUnits=kg/(m^3)  GraphicType=FromGeometry  MarkerShape=Sphere  MarkerSize=10  MarkerSizeUnits=m  GraphicVisPropType=SimpleVisualProperties  GraphicDiffuseColor=[0.5 0.5 0.5]  GraphicSpecularColor=[0.5 0.5 0.5 1.0]  GraphicAmbientColor=[0.15 0.15 0.15 1.0]  GraphicEmissiveColor=[0.0 0.0 0.0 1.0]  GraphicShininess=75  GraphicOpacity=1.0  GeometryShape=FromFile  RectangleSize=[1 1]  RectangleSizeUnits=m  BrickDimensions=[1 1 1]  BrickDimensionUnits=m  CylinderRadius=1  CylinderRadiusUnits=m  CylinderLength=1  CylinderLengthUnits=m  SphereRadius=1  SphereRadiusUnits=m  EllipsoidRadii=[1 1 1]  EllipsoidRadiiUnits=m  ExtrusionCrossSection=[1 1; -1 1; -1 -1; 1 -1]  ExtrusionCrossSectionUnits=m  ExtrusionLength=1  ExtrusionLengthUnits=m  PolygonNumSides=3  PolygonOuterRadius=1  PolygonOuterRadiusUnits=m  ExtGeomFileType=STL  ExtGeomFileName=D:\Ker Lann\systemes\darwin\kinematics\STL\Right_Thigh.STL  ExtGeomFileUnits=mm  RevolutionCrossSection=[1 1; 1 -1; 2 -1; 2 1]  RevolutionCrossSectionUnits=m  RevolutionExtent=Full  RevolutionAngle=180  RevolutionAngleUnits=deg  BlockFunction=simmechanics.library.body_elements.solid
  Right Hip Pitch : PMIOPort  Port=1  Side=Left
  Right Knee : PMIOPort  Port=2  Side=Right
  connections:
  Right Hip Pitch Axis to Right Lower Leg Base/LConn1 -- Right Hip Pitch/RConn1 -- Solid/RConn1
  Right Knee/RConn1 -- Right Hip Pitch Axis to Right Lower Leg Base/RConn1

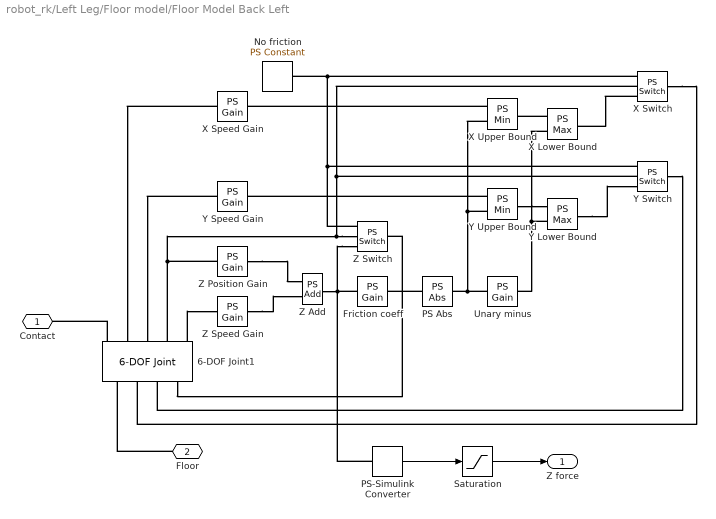
== system robot_rk/Left Leg/Floor model/Floor Model Back Left ==
  6-DOF Joint1 : sm_lib/Joints/6-DOF Joint  SenseConstraintForce=off  SenseConstraintForceX=off  SenseConstraintForceY=off  SenseConstraintForceZ=off  SenseConstraintTorque=off  SenseConstraintTorqueX=off  SenseConstraintTorqueY=off  SenseConstraintTorqueZ=off  SenseTotalForce=off  SenseTotalForceX=off  SenseTotalForceY=off  SenseTotalForceZ=off  SenseTotalTorque=off  SenseTotalTorqueX=off  SenseTotalTorqueY=off  SenseTotalTorqueZ=off  CompositeWrenchDir=FollowerOnBase  CompositeWrenchFrame=BaseFrame  PxEquilibriumPosition=0  PxEquilibriumPositionUnits=m  PxSpringStiffness=0  PxSpringStiffnessUnits=N/m  PxDampingCoefficient=0  PxDampingCoefficientUnits=N/(m/s)  PxTorqueActuationMode=InputTorque  PxMotionActuationMode=ComputedMotion  PxSensePosition=off  PxSenseVelocity=on  PxSenseAcceleration=off  PxSenseTorqueForce=off  PxPositionTargetValue=0  PxPositionTargetValueUnits=m  PxPositionTargetSpecify=off  PxPositionTargetPriority=High  PxVelocityTargetValue=0  PxVelocityTargetValueUnits=m/s  PxVelocityTargetSpecify=off  PxVelocityTargetPriority=High  PyEquilibriumPosition=0  PyEquilibriumPositionUnits=m  PySpringStiffness=0  PySpringStiffnessUnits=N/m  PyDampingCoefficient=0  PyDampingCoefficientUnits=N/(m/s)  PyTorqueActuationMode=InputTorque  PyMotionActuationMode=ComputedMotion  PySensePosition=off  PySenseVelocity=on  PySenseAcceleration=off  PySenseTorqueForce=off  PyPositionTargetValue=0  PyPositionTargetValueUnits=m  PyPositionTargetSpecify=off  PyPositionTargetPriority=High  PyVelocityTargetValue=0  PyVelocityTargetValueUnits=m/s  PyVelocityTargetSpecify=off  PyVelocityTargetPriority=High  PzEquilibriumPosition=0  PzEquilibriumPositionUnits=m  PzSpringStiffness=0  PzSpringStiffnessUnits=N/m  PzDampingCoefficient=0  PzDampingCoefficientUnits=N/(m/s)  PzTorqueActuationMode=InputTorque  PzMotionActuationMode=ComputedMotion  PzSensePosition=on  PzSenseVelocity=on  PzSenseAcceleration=off  PzSenseTorqueForce=off  PzPositionTargetValue=0  PzPositionTargetValueUnits=m  PzPositionTargetSpecify=off  PzPositionTargetPriority=High  PzVelocityTargetValue=0  PzVelocityTargetValueUnits=m/s  PzVelocityTargetSpecify=off  PzVelocityTargetPriority=High  SphDefPosRotationMethod=None  SphDefPosRotationAngleUnits=deg  SphDefPosRotationStandardAxis=+Z  SphDefPosRotationAngle=0.0  SphDefPosRotationArbitraryAxis=[0 0 1]  SphDefPosFollAlignAxisA=+X  SphDefPosBaseAlignAxisA=+Y  SphDefPosFollAlignAxisB=+Y  SphDefPosBaseAlignAxisB=+Z  SphDefPosRotationMatrix=[1 0 0; 0 1 0; 0 0 1]  SphEqPosRotationMethod=None  SphEqPosRotationAngleUnits=deg  SphEqPosRotationStandardAxis=+Z  SphEqPosRotationAngle=0.0  SphEqPosRotationArbitraryAxis=[0 0 1]  SphEqPosFollAlignAxisA=+X  SphEqPosBaseAlignAxisA=+Y  SphEqPosFollAlignAxisB=+Y  SphEqPosBaseAlignAxisB=+Z  SphEqPosRotationMatrix=[1 0 0; 0 1 0; 0 0 1]  SphSpringStiffness=0  SphSpringStiffnessUnits=N*m/deg  SphDampingCoefficient=0  SphDampingCoefficientUnits=N*m/(deg/s)  SphActuateTorqueX=off  SphActuateTorqueY=off  SphActuateTorqueZ=off  SphActuateTorque=off  SphTorqueActuationMode=NoTorque  SphMotionActuationMode=ComputedMotion  SphActuationFrame=BaseFrame  SphSensePosition=off  SphSenseVelocityX=off  SphSenseVelocityY=off  SphSenseVelocityZ=off  SphSenseVelocity=off  SphSenseAccelerationX=off  SphSenseAccelerationY=off  SphSenseAccelerationZ=off  SphSenseAcceleration=off  SphSenseTorqueX=off  SphSenseTorqueY=off  SphSenseTorqueZ=off  SphSenseTorqueForce=off  SphSensingFrame=BaseFrame  SphPositionTargetRotationMethod=None  SphPositionTargetRotationAngleUnits=deg  SphPositionTargetRotationStandardAxis=+Z  SphPositionTargetRotationAngle=0.0  SphPositionTargetRotationArbitraryAxis=[0 0 1]  SphPositionTargetFollAlignAxisA=+X  SphPositionTargetBaseAlignAxisA=+Y  SphPositionTargetFollAlignAxisB=+Y  SphPositionTargetBaseAlignAxisB=+Z  SphPositionTargetRotationMatrix=[1 0 0; 0 1 0; 0 0 1]  SphPositionTargetSpecify=off  SphPositionTargetPriority=High  SphVelocityTargetValue=[0 0 0]  SphVelocityTargetValueUnits=deg/s  SphVelocityTargetSpecify=off  SphVelocityTargetPriority=High  SphVelocityTargetInFollowerFrame=on  BlockFunction=simmechanics.library.joints.sixdof_joint
  Friction coeff : fl_lib/Physical Signals/Functions/PS Gain  gain=robot_floor_friction_coeff
  No friction : fl_lib/Physical Signals/Sources/PS Constant  constant=0
  PS Abs : fl_lib/Physical Signals/Nonlinear Operators/PS Abs
  PS-Simulink Converter : nesl_utility/PS-Simulink Converter  PhysicalDomain=network_engine_domain  SubClassName=ps_output  LeftPortType=input  RightPortType=output  PseudoPeriodic=off  Frequencies=[]  Unit=N  AffineConversion=off
  Saturation : Saturate  UpperLimit=+inf  LowerLimit=0
  Unary minus : fl_lib/Physical Signals/Functions/PS Gain  gain=-1
  X Lower Bound : fl_lib/Physical Signals/Nonlinear Operators/PS Max
  X Speed Gain : fl_lib/Physical Signals/Functions/PS Gain  gain=robot_floor_speed_gain
  X Switch : fl_lib/Physical Signals/Nonlinear Operators/PS Switch  Threshold=0
  X Upper Bound : fl_lib/Physical Signals/Nonlinear Operators/PS Min
  Y Lower Bound : fl_lib/Physical Signals/Nonlinear Operators/PS Max
  Y Speed Gain : fl_lib/Physical Signals/Functions/PS Gain  gain=robot_floor_speed_gain
  Y Switch : fl_lib/Physical Signals/Nonlinear Operators/PS Switch  Threshold=0
  Y Upper Bound : fl_lib/Physical Signals/Nonlinear Operators/PS Min
  Z Add : fl_lib/Physical Signals/Functions/PS Add
  Z Position Gain : fl_lib/Physical Signals/Functions/PS Gain  gain=robot_floor_position_gain
  Z Speed Gain : fl_lib/Physical Signals/Functions/PS Gain  gain=robot_floor_speed_gain
  Z Switch : fl_lib/Physical Signals/Nonlinear Operators/PS Switch  Threshold=0
  Contact : PMIOPort  Port=1  Side=Left
  Floor : PMIOPort  Port=2  Side=Right
  Z force : Outport
  wires:
  PS-Simulink Converter/1 -> Saturation/1
  Saturation/1 -> Z force/1
  connections:
  Floor/RConn1 -- 6-DOF Joint1/LConn1
  6-DOF Joint1/RConn1 -- Contact/RConn1
  No friction/RConn1 -- Y Switch/LConn1 -- Z Switch/LConn1 -- X Switch/LConn1
  Z Position Gain/RConn1 -- Z Add/LConn1
  Z Switch/LConn3 -- Z Add/RConn1 -- Friction coeff/LConn1 -- PS-Simulink Converter/LConn1
  Z Speed Gain/RConn1 -- Z Add/LConn2
  6-DOF Joint1/RConn5 -- Z Speed Gain/LConn1
  6-DOF Joint1/LConn4 -- Z Switch/RConn1
  Z Switch/LConn2 -- Z Position Gain/LConn1 -- 6-DOF Joint1/RConn4 -- X Switch/LConn2 -- Y Switch/LConn2
  Y Switch/RConn1 -- 6-DOF Joint1/LConn3
  Y Speed Gain/LConn1 -- 6-DOF Joint1/RConn3
  PS Abs/LConn1 -- Friction coeff/RConn1
  PS Abs/RConn1 -- Unary minus/LConn1 -- X Upper Bound/LConn2 -- Y Upper Bound/LConn2
  Y Upper Bound/RConn1 -- Y Lower Bound/LConn1
  Y Lower Bound/LConn2 -- Unary minus/RConn1 -- X Lower Bound/LConn2
  Y Lower Bound/RConn1 -- Y Switch/LConn3
  Y Upper Bound/LConn1 -- Y Speed Gain/RConn1
  X Speed Gain/LConn1 -- 6-DOF Joint1/RConn2
  X Upper Bound/LConn1 -- X Speed Gain/RConn1
  X Lower Bound/LConn1 -- X Upper Bound/RConn1
  X Switch/LConn3 -- X Lower Bound/RConn1
  X Switch/RConn1 -- 6-DOF Joint1/LConn2
